simulink model "linedetectenew"  (R2018b)
settings: Solver=FixedStepDiscrete  StartTime=0.0  StopTime=0  FixedStep=0.2  RelTol=1e-3
undefined symbols (not defined in the file or in its folder): gray, Rec, SDTV
libraries: visiontransforms x2, embdlinuxlib x2, androidaudiovideolib x1, visionconversions x1, visiontextngfix x1, visionanalysis x1, visionstatistics x1, visionsources x1
settings Model: Creator=Simon  LastModifiedBy=chada

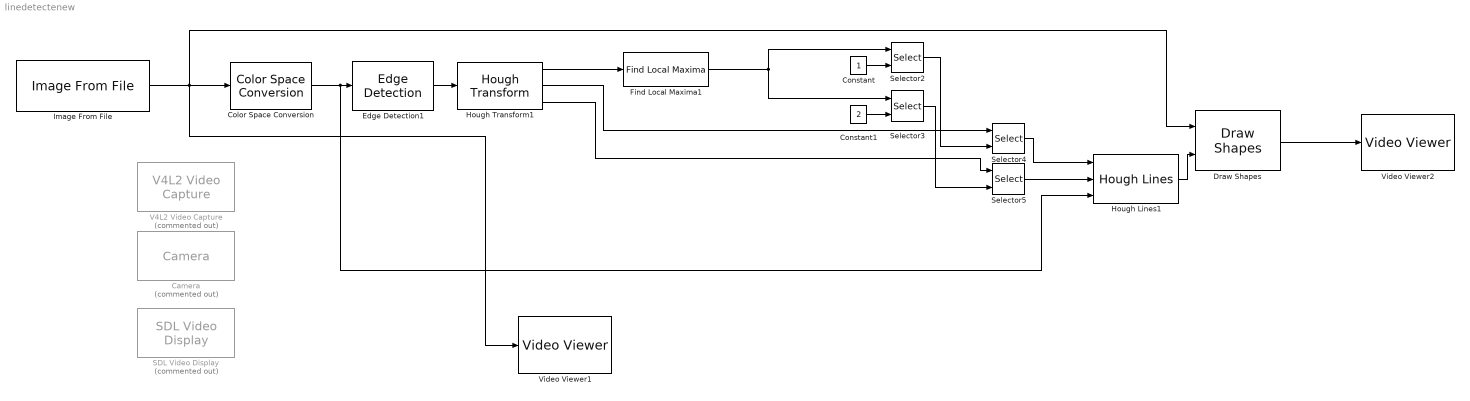
== system linedetectenew ==
  Camera : androidaudiovideolib/Camera  Commented=on  CameraLocation=Back  CameraResolutions=Back - 640x480  Width=640  Height=480  SampleTime=0.1  BlockPlatform=Android
      settings: SourceProductName=Simulink Support Package for Android Devices  SourceProductBaseCode=ANDROID
  Color Space Conversion : visionconversions/Color Space  Conversion  conversion=Obsolete  conversionActive=R'G'B' to intensity  wp_str=D65  rec=Rec. 601 (SDTV)  sys=1125/60/2:1  imagePorts=One multidimensional signal
      settings: SourceProductName=Computer Vision System Toolbox
  Constant : Constant
  Constant1 : Constant  Value=2
  Draw Shapes : visiontextngfix/Draw Shapes  shape=Lines  fill=off  lineWidth=5  fillClrSource=Specify via dialog  display=User-specified value  intensity=200  color=[255 000 0]  opacity=0.6  viewport=Entire image  antialiasing=off  inType=Obsolete  imagePorts=One multidimensional signal  prodOutputMode=Binary point scaling  prodOutputWordLength=32  prodOutputFracLength=14  memoryMode=Specify word length  memoryWordLength=16  memoryFracLength=14  roundingMode=Floor  overflowMode=off
      settings: SourceProductName=Computer Vision System Toolbox
  Edge Detection1 : visionanalysis/Edge Detection  method=Sobel  outputType=Binary image  userDefinedThreshold=off  thresholdSource=Input port  threshold=20  thresholdTuning=4  edgeThinning=off  threshold_canny=[0.25 0.60]  autoPercent=70  sigma=1  roundingMode=Floor  overflowMode=off  prodOutputMode=Binary point scaling  prodOutputWordLength=32  prodOutputFracLength=8  prodOutputSlope=2^-8  accumSlope=2^-8  outputSlope=2^-4
      settings: SourceProductName=Computer Vision System Toolbox  SourceProductBaseCode=VP
  Find Local Maxima1 : visionstatistics/Find Local Maxima  num_peaks=1  nhood_size=[5 7]  src_thresh=Obsolete9b  src_thresh_inuse=Specify via dialog  threshold=10  inputIsHough=on  dt_peak=uint32  isOutVarDim=on  dt_count=uint32
      settings: SourceProductName=Computer Vision System Toolbox  SourceProductBaseCode=VP
  Hough Lines1 : visiontransforms/Hough Lines  sineCompMethod=Trigonometric function  thetaRes=pi/180  firstCoeffMode=Specify word length  firstCoeffWordLength=16  firstCoeffFracLength=15  prodOutputMode=Binary point scaling  prodOutputWordLength=32  prodOutputFracLength=16  roundingMode=Nearest  overflowMode=on
      settings: SourceProductName=Computer Vision System Toolbox  SourceProductBaseCode=VP
  Hough Transform1 : visiontransforms/Hough Transform  theta_res=pi/360  rho_res=1  out_theta_rho=on  outdtmode=double  roundingMode=Nearest  overflowMode=on  firstCoeffMode=Binary point scaling  firstCoeffWordLength=16  firstCoeffFracLength=14  firstCoeffSlope=2^-14  secondCoeffMode=Binary point scaling  secondCoeffWordLength=32  secondCoeffFracLength=16  secondCoeffSlope=2^-16  prodOutputMode=Binary point scaling  prodOutputWordLength=32  prodOutputFracLength=20  prodOutputSlope=2^-20  accumMode=Binary point scaling  accumWordLength=32  accumFracLength=20  accumSlope=2^-20  outputMode=Binary point scaling  outputWordLength=16  outputFracLength=0  outputSlope=2^0  memoryMode=Binary point scaling  memoryWordLength=32  memoryFracLength=16  memorySlope=2^-16
      settings: SourceProductName=Computer Vision System Toolbox  SourceProductBaseCode=VP
  Image From File : visionsources/Image From File  Tag=vipblks_nd  FileName=C:\Users\chada\Downloads\62189695_465650710869758_3509252219457241088_n.jpg  imagePorts=One multidimensional signal  Ts=0  ImageDataType=Inherit from input image  Signed=on  WordLength=16  sdImageDataType=uint(8)  FractionLengthMode=User-defined  FractionLength=15  OutPortLabels=R|G|B
      settings: SourceProductName=Computer Vision System Toolbox
  SDL Video Display : embdlinuxlib/SDL Video Display  Commented=on  pixelFormat=RGB  pixelOrder=Planar  rowMajor=on  blockPlatform=Raspberry Pi
      settings: SourceProductName=Simulink Support Package for Raspberry Pi Hardware  SourceProductBaseCode=RASPPI
  Selector2 : Selector  InputPortWidth=2  IndexOptions=Index vector (port)  Indices=1  OutputSizes=1
  Selector3 : Selector  InputPortWidth=2  IndexOptions=Index vector (port)  Indices=0  OutputSizes=1
  Selector4 : Selector  InputPortWidth=360  IndexOptions=Index vector (port)  Indices=[1 3]  OutputSizes=1
  Selector5 : Selector  InputPortWidth=1199  IndexOptions=Index vector (port)  Indices=[1 3]  OutputSizes=1
  V4L2 Video Capture : embdlinuxlib/V4L2 Video Capture  Commented=on  m_devName='/dev/video0'  roi=[0, 0, 640, 480]  imSizeSelection=320x240  imSize=[640, 480]  pixelFormat=RGB  pixelOrder=Planar  sampleTime=1/4  simOutput=Colorbars  blockPlatform=Raspberry Pi
      settings: SourceProductName=Simulink Support Package for Raspberry Pi Hardware  SourceProductBaseCode=RASPPI
  Video Viewer1 : VideoViewer  colormapValue=gray(256)  FigPos=[-31 846 728 591]
  Video Viewer2 : VideoViewer  colormapValue=gray(256)  FigPos=[733 852 662 627]
  wires:
  Constant1/1 -> Selector3/2
  Hough Lines1/1 -> Draw Shapes/2
  Selector5/1 -> Hough Lines1/2
  Find Local Maxima1/1 -> Selector2/1, Selector3/1
  Draw Shapes/1 -> Video Viewer2/1
  Hough Transform1/3 -> Selector5/1
  Hough Transform1/2 -> Selector4/1
  Hough Transform1/1 -> Find Local Maxima1/1
  Edge Detection1/1 -> Hough Transform1/1
  Color Space Conversion/1 -> Hough Lines1/3, Edge Detection1/1
  Selector2/1 -> Selector4/2
  Selector3/1 -> Selector5/2
  Constant/1 -> Selector2/2
  Selector4/1 -> Hough Lines1/1
  Image From File/1 -> Video Viewer1/1, Draw Shapes/1, Color Space Conversion/1
